simulink model "mud"  (Simulink 6.0)
settings: Solver=ode45  StartTime=0.0  StopTime=5000.0  RelTol=1e-3
undefined symbols (not defined in the file or in its folder): cputime
libraries: commsink2 x3
settings Model: LastModifiedBy=god

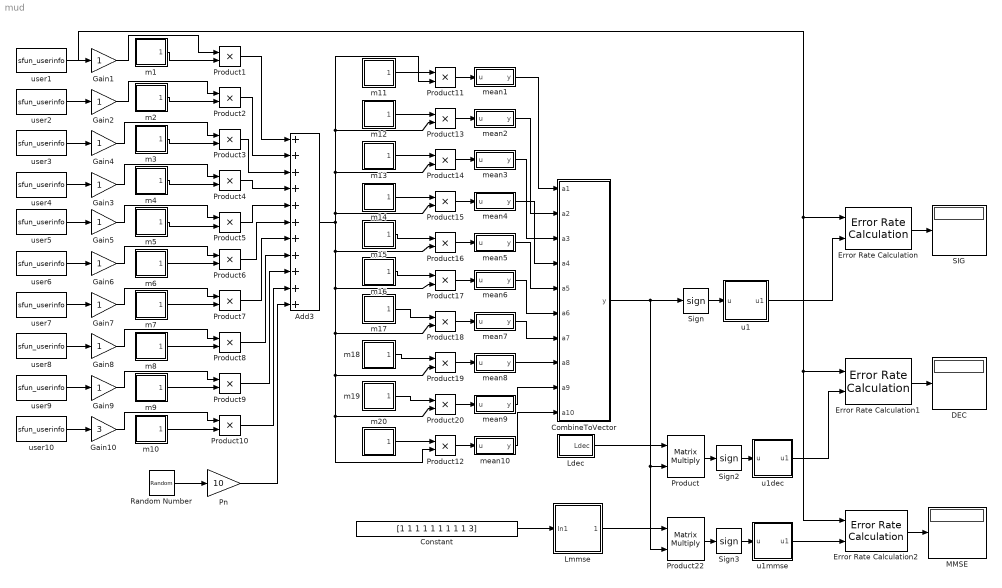
== system mud ==
  Add3 : Sum  Inputs=+++++++++++  OutScaling=2^-10  SampleTime=1
  CombineToVector : Stateflow chart
  Constant : Constant  Value=[1 1 1 1 1 1 1 1 1 3]
  DEC : Display
  Error Rate Calculation : commsink2/Error Rate Calculation  N=0  st_delay=0  cp_mode=Entire frame  subframe=[]  PMode=Port  WsName=ErrorVec  RsMode2=off  stop=off  numErr=100  maxBits=1e6
  Error Rate Calculation1 : commsink2/Error Rate Calculation  N=0  st_delay=0  cp_mode=Entire frame  subframe=[]  PMode=Port  WsName=ErrorVec  RsMode2=off  stop=off  numErr=100  maxBits=1e6
  Error Rate Calculation2 : commsink2/Error Rate Calculation  N=0  st_delay=0  cp_mode=Entire frame  subframe=[]  PMode=Port  WsName=ErrorVec  RsMode2=off  stop=off  numErr=100  maxBits=1e6
  Gain{1..9} (9 alike) : Gain  SampleTime=1
  Gain10 : Gain  Gain=3  SampleTime=1
  Ldec : Subsystem
  Lmmse : Subsystem
  MMSE : Display
  Pn : Gain  Gain=10  SampleTime=1
  Product : Product  Multiplication=Matrix(*)  RndMeth=Zero
  Product{1..20} (20 alike) : Product  SampleTime=1  RndMeth=Zero
  Product22 : Product  Multiplication=Matrix(*)  RndMeth=Zero
  Random Number : RandomNumber  Seed=cputime  SampleTime=1
  SIG : Display
  Sign : Signum
  Sign2 : Signum
  Sign3 : Signum
  m1 : Subsystem
  m10 : Subsystem
  m11 : Subsystem
  m12 : Subsystem
  m13 : Subsystem
  m14 : Subsystem
  m15 : Subsystem
  m16 : Subsystem
  m17 : Subsystem
  m18 : Subsystem
  m19 : Subsystem
  m2 : Subsystem
  m20 : Subsystem
  m3 : Subsystem
  m4 : Subsystem
  m5 : Subsystem
  m6 : Subsystem
  m7 : Subsystem
  m8 : Subsystem
  m9 : Subsystem
  mean1 : Stateflow chart
  mean10 : Stateflow chart
  mean2 : Stateflow chart
  mean3 : Stateflow chart
  mean4 : Stateflow chart
  mean5 : Stateflow chart
  mean6 : Stateflow chart
  mean7 : Stateflow chart
  mean8 : Stateflow chart
  mean9 : Stateflow chart
  u1 : Stateflow chart
  u1dec : Stateflow chart
  u1mmse : Stateflow chart
  user{1..10} (10 alike) : S-Function  FunctionName=sfun_userinfo
  wires:
  Gain1/1 -> Product1/1
  m1/1(Out1) -> Product1/2
  Gain2/1 -> Product2/1
  m2/1(Out1) -> Product2/2
  Gain4/1 -> Product3/1
  m3/1(Out1) -> Product3/2
  Gain3/1 -> Product4/1
  m4/1(Out1) -> Product4/2
  Gain5/1 -> Product5/1
  m5/1(Out1) -> Product5/2
  Gain6/1 -> Product6/1
  m6/1(Out1) -> Product6/2
  Gain7/1 -> Product7/1
  m7/1(Out1) -> Product7/2
  Gain8/1 -> Product8/1
  m8/1(Out1) -> Product8/2
  Gain9/1 -> Product9/1
  m9/1(Out1) -> Product9/2
  Gain10/1 -> Product10/1
  m10/1(Out1) -> Product10/2
  Random Number/1 -> Pn/1
  m11/1(Out1) -> Product11/1
  m12/1(Out1) -> Product13/1
  m13/1(Out1) -> Product14/1
  m14/1(Out1) -> Product15/1
  m15/1(Out1) -> Product16/1
  m16/1(Out1) -> Product17/1
  m17/1(Out1) -> Product18/1
  m18/1(Out1) -> Product19/1
  m20/1(Out1) -> Product12/1
  Add3/1 -> Product11/2, Product13/2, Product14/2, Product15/2, Product16/2, Product17/2, Product18/2, Product19/2, Product12/2, Product20/2
  Product13/1 -> mean2/1(u)
  Product14/1 -> mean3/1(u)
  Product15/1 -> mean4/1(u)
  Product16/1 -> mean5/1(u)
  Product17/1 -> mean6/1(u)
  Product18/1 -> mean7/1(u)
  Product19/1 -> mean8/1(u)
  Product20/1 -> mean9/1(u)
  Product12/1 -> mean10/1(u)
  Product11/1 -> mean1/1(u)
  mean1/1(y) -> CombineToVector/1(a1)
  mean2/1(y) -> CombineToVector/2(a2)
  mean3/1(y) -> CombineToVector/3(a3)
  mean4/1(y) -> CombineToVector/4(a4)
  mean5/1(y) -> CombineToVector/5(a5)
  mean6/1(y) -> CombineToVector/6(a6)
  mean7/1(y) -> CombineToVector/7(a7)
  mean9/1(y) -> CombineToVector/9(a9)
  mean10/1(y) -> CombineToVector/10(a10)
  CombineToVector/1(y) -> Product/2, Product22/2, Sign/1
  mean8/1(y) -> CombineToVector/8(a8)
  Product/1 -> Sign2/1
  user1/1 -> Gain1/1, Error Rate Calculation/1, Error Rate Calculation1/1, Error Rate Calculation2/1
  user2/1 -> Gain2/1
  user3/1 -> Gain4/1
  user4/1 -> Gain3/1
  user5/1 -> Gain5/1
  user6/1 -> Gain6/1
  user7/1 -> Gain7/1
  user8/1 -> Gain8/1
  user10/1 -> Gain10/1
  user9/1 -> Gain9/1
  Error Rate Calculation1/1 -> DEC/1
  Sign/1 -> u1/1(u)
  Sign2/1 -> u1dec/1(u)
  Sign3/1 -> u1mmse/1(u)
  u1/1(u1) -> Error Rate Calculation/2
  Product1/1 -> Add3/1
  Product2/1 -> Add3/2
  Product3/1 -> Add3/3
  Product4/1 -> Add3/4
  Product5/1 -> Add3/5
  Product6/1 -> Add3/6
  Product9/1 -> Add3/9
  Product10/1 -> Add3/10
  Product7/1 -> Add3/7
  Product8/1 -> Add3/8
  m19/1(Out1) -> Product20/1
  Product22/1 -> Sign3/1
  u1mmse/1(u1) -> Error Rate Calculation2/2
  u1dec/1(u1) -> Error Rate Calculation1/2
  Error Rate Calculation2/1 -> MMSE/1
  Error Rate Calculation/1 -> SIG/1
  Constant/1 -> Lmmse/1(In1)
  Lmmse/1(Lmmse) -> Product22/1
  Ldec/1(Ldec) -> Product/1
  Pn/1 -> Add3/11

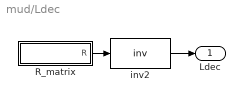
== system mud/Ldec ==
  R_matrix : Stateflow chart
  inv2 : MATLABFcn  MATLABFcn=inv  Output1D=off
  Ldec : Outport
  wires:
  R_matrix/1(R) -> inv2/1
  inv2/1 -> Ldec/1

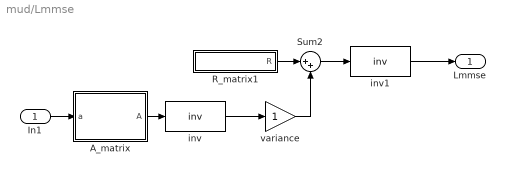
== system mud/Lmmse ==
  In1 : Inport  Port=1  LatchInput=off
  A_matrix : Stateflow chart
  R_matrix1 : Stateflow chart
  Sum2 : Sum  Inputs=|++
  inv : MATLABFcn  MATLABFcn=inv  Output1D=off
  inv1 : MATLABFcn  MATLABFcn=inv  Output1D=off
  variance : Gain
  Lmmse : Outport
  wires:
  A_matrix/1(A) -> inv/1
  inv/1 -> variance/1
  R_matrix1/1(R) -> Sum2/1
  variance/1 -> Sum2/2
  Sum2/1 -> inv1/1
  inv1/1 -> Lmmse/1
  In1/1 -> A_matrix/1(a)

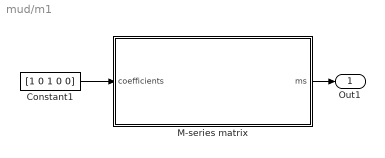
== system mud/m1 ==
  Constant1 : Constant  Value=[1 0 1 0 0]
  M-series matrix : Stateflow chart
  Out1 : Outport
  wires:
  Constant1/1 -> M-series matrix/1(coefficients)
  M-series matrix/1(ms) -> Out1/1

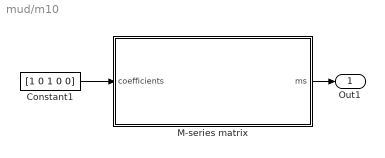
== system mud/m10 ==
  Constant1 : Constant  Value=[1 0 1 0 0]
  M-series matrix : Stateflow chart
  Out1 : Outport
  wires:
  Constant1/1 -> M-series matrix/1(coefficients)
  M-series matrix/1(ms) -> Out1/1

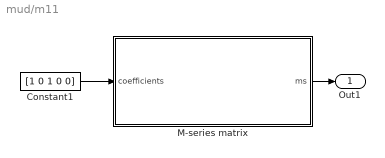
== system mud/m11 ==
  Constant1 : Constant  Value=[1 0 1 0 0]
  M-series matrix : Stateflow chart
  Out1 : Outport
  wires:
  M-series matrix/1(ms) -> Out1/1
  Constant1/1 -> M-series matrix/1(coefficients)

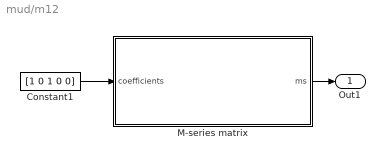
== system mud/m12 ==
  Constant1 : Constant  Value=[1 0 1 0 0]
  M-series matrix : Stateflow chart
  Out1 : Outport
  wires:
  M-series matrix/1(ms) -> Out1/1
  Constant1/1 -> M-series matrix/1(coefficients)

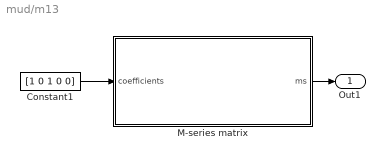
== system mud/m13 ==
  Constant1 : Constant  Value=[1 0 1 0 0]
  M-series matrix : Stateflow chart
  Out1 : Outport
  wires:
  M-series matrix/1(ms) -> Out1/1
  Constant1/1 -> M-series matrix/1(coefficients)

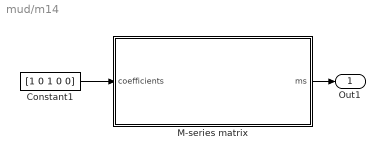
== system mud/m14 ==
  Constant1 : Constant  Value=[1 0 1 0 0]
  M-series matrix : Stateflow chart
  Out1 : Outport
  wires:
  M-series matrix/1(ms) -> Out1/1
  Constant1/1 -> M-series matrix/1(coefficients)

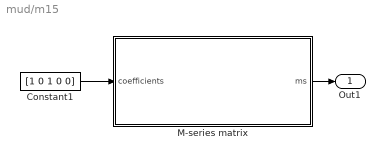
== system mud/m15 ==
  Constant1 : Constant  Value=[1 0 1 0 0]
  M-series matrix : Stateflow chart
  Out1 : Outport
  wires:
  M-series matrix/1(ms) -> Out1/1
  Constant1/1 -> M-series matrix/1(coefficients)

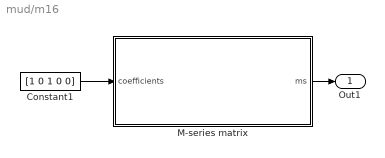
== system mud/m16 ==
  Constant1 : Constant  Value=[1 0 1 0 0]
  M-series matrix : Stateflow chart
  Out1 : Outport
  wires:
  M-series matrix/1(ms) -> Out1/1
  Constant1/1 -> M-series matrix/1(coefficients)

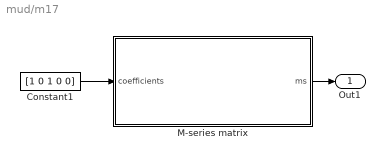
== system mud/m17 ==
  Constant1 : Constant  Value=[1 0 1 0 0]
  M-series matrix : Stateflow chart
  Out1 : Outport
  wires:
  M-series matrix/1(ms) -> Out1/1
  Constant1/1 -> M-series matrix/1(coefficients)

== system mud/m18 ==
  Constant1 : Constant  Value=[1 0 1 0 0]
  M-series matrix : Stateflow chart
  Out1 : Outport
  wires:
  M-series matrix/1(ms) -> Out1/1
  Constant1/1 -> M-series matrix/1(coefficients)

== system mud/m19 ==
  Constant1 : Constant  Value=[1 0 1 0 0]
  M-series matrix : Stateflow chart
  Out1 : Outport
  wires:
  M-series matrix/1(ms) -> Out1/1
  Constant1/1 -> M-series matrix/1(coefficients)

== system mud/m2 ==
  Constant1 : Constant  Value=[1 0 1 0 0]
  M-series matrix : Stateflow chart
  Out1 : Outport
  wires:
  Constant1/1 -> M-series matrix/1(coefficients)
  M-series matrix/1(ms) -> Out1/1

== system mud/m20 ==
  Constant1 : Constant  Value=[1 0 1 0 0]
  M-series matrix : Stateflow chart
  Out1 : Outport
  wires:
  M-series matrix/1(ms) -> Out1/1
  Constant1/1 -> M-series matrix/1(coefficients)

== system mud/m3 ==
  Constant1 : Constant  Value=[1 0 1 0 0]
  M-series matrix : Stateflow chart
  Out1 : Outport
  wires:
  Constant1/1 -> M-series matrix/1(coefficients)
  M-series matrix/1(ms) -> Out1/1

== system mud/m4 ==
  Constant1 : Constant  Value=[1 0 1 0 0]
  M-series matrix : Stateflow chart
  Out1 : Outport
  wires:
  Constant1/1 -> M-series matrix/1(coefficients)
  M-series matrix/1(ms) -> Out1/1

== system mud/m5 ==
  Constant1 : Constant  Value=[1 0 1 0 0]
  M-series matrix : Stateflow chart
  Out1 : Outport
  wires:
  Constant1/1 -> M-series matrix/1(coefficients)
  M-series matrix/1(ms) -> Out1/1

== system mud/m6 ==
  Constant1 : Constant  Value=[1 0 1 0 0]
  M-series matrix : Stateflow chart
  Out1 : Outport
  wires:
  Constant1/1 -> M-series matrix/1(coefficients)
  M-series matrix/1(ms) -> Out1/1

== system mud/m7 ==
  Constant1 : Constant  Value=[1 0 1 0 0]
  M-series matrix : Stateflow chart
  Out1 : Outport
  wires:
  Constant1/1 -> M-series matrix/1(coefficients)
  M-series matrix/1(ms) -> Out1/1

== system mud/m8 ==
  Constant1 : Constant  Value=[1 0 1 0 0]
  M-series matrix : Stateflow chart
  Out1 : Outport
  wires:
  Constant1/1 -> M-series matrix/1(coefficients)
  M-series matrix/1(ms) -> Out1/1

== system mud/m9 ==
  Constant1 : Constant  Value=[1 0 1 0 0]
  M-series matrix : Stateflow chart
  Out1 : Outport
  wires:
  Constant1/1 -> M-series matrix/1(coefficients)
  M-series matrix/1(ms) -> Out1/1

== matlab function m2/M-series matrix ==
  data: coefficients input inherited; ms output inherited
function ms = mseries(coefficients)
len=length(coefficients);
L=2^len-1;
registers=[zeros(1,len-1),1];
newregisters=zeros(1,len);
a=[0 0 0 0 0 0 0 0 0 0 0 0 0 0 0 0 0 0 0 0 0 0 0 0 0 0 0 0 0 0 0];
a(1)=registers(1);
for i= 2:L
    newregisters(1:len-1) = registers(2:len);
    newregisters(len) = mod(sum(coefficients.*registers'),2);
    registers=newregisters;
    a(i)=registers(1);
end
for j=1:L
    if a(j)==0
        a(j)=1;
    else
        a(j)=-1;
    end
end

atemp=zeros(31);
for p=1:L
  atemp(p,:)=a;
  temp=a(1);
  for q=1:L-1
  a(q)=a(q+1);
  end
  a(L)=temp;
end
ms=atemp(2,:);

== matlab function m3/M-series matrix ==
  data: coefficients input inherited; ms output inherited
function ms = mseries(coefficients)
len=length(coefficients);
L=2^len-1;
registers=[zeros(1,len-1),1];
newregisters=zeros(1,len);
a=[0 0 0 0 0 0 0 0 0 0 0 0 0 0 0 0 0 0 0 0 0 0 0 0 0 0 0 0 0 0 0];
a(1)=registers(1);
for i= 2:L
    newregisters(1:len-1) = registers(2:len);
    newregisters(len) = mod(sum(coefficients.*registers'),2);
    registers=newregisters;
    a(i)=registers(1);
end
for j=1:L
    if a(j)==0
        a(j)=1;
    else
        a(j)=-1;
    end
end

atemp=zeros(31);
for p=1:L
  atemp(p,:)=a;
  temp=a(1);
  for q=1:L-1
  a(q)=a(q+1);
  end
  a(L)=temp;
end
ms=atemp(3,:);

== matlab function m4/M-series matrix ==
  data: coefficients input inherited; ms output inherited
function ms = mseries(coefficients)
len=length(coefficients);
L=2^len-1;
registers=[zeros(1,len-1),1];
newregisters=zeros(1,len);
a=[0 0 0 0 0 0 0 0 0 0 0 0 0 0 0 0 0 0 0 0 0 0 0 0 0 0 0 0 0 0 0];
a(1)=registers(1);
for i= 2:L
    newregisters(1:len-1) = registers(2:len);
    newregisters(len) = mod(sum(coefficients.*registers'),2);
    registers=newregisters;
    a(i)=registers(1);
end
for j=1:L
    if a(j)==0
        a(j)=1;
    else
        a(j)=-1;
    end
end

atemp=zeros(31);
for p=1:L
  atemp(p,:)=a;
  temp=a(1);
  for q=1:L-1
  a(q)=a(q+1);
  end
  a(L)=temp;
end
ms=atemp(4,:);

== matlab function m5/M-series matrix ==
  data: coefficients input inherited; ms output inherited
function ms = mseries(coefficients)
len=length(coefficients);
L=2^len-1;
registers=[zeros(1,len-1),1];
newregisters=zeros(1,len);
a=[0 0 0 0 0 0 0 0 0 0 0 0 0 0 0 0 0 0 0 0 0 0 0 0 0 0 0 0 0 0 0];
a(1)=registers(1);
for i= 2:L
    newregisters(1:len-1) = registers(2:len);
    newregisters(len) = mod(sum(coefficients.*registers'),2);
    registers=newregisters;
    a(i)=registers(1);
end
for j=1:L
    if a(j)==0
        a(j)=1;
    else
        a(j)=-1;
    end
end

atemp=zeros(31);
for p=1:L
  atemp(p,:)=a;
  temp=a(1);
  for q=1:L-1
  a(q)=a(q+1);
  end
  a(L)=temp;
end
ms=atemp(5,:);

== matlab function m6/M-series matrix ==
  data: coefficients input inherited; ms output inherited
function ms = mseries(coefficients)
len=length(coefficients);
L=2^len-1;
registers=[zeros(1,len-1),1];
newregisters=zeros(1,len);
a=[0 0 0 0 0 0 0 0 0 0 0 0 0 0 0 0 0 0 0 0 0 0 0 0 0 0 0 0 0 0 0];
a(1)=registers(1);
for i= 2:L
    newregisters(1:len-1) = registers(2:len);
    newregisters(len) = mod(sum(coefficients.*registers'),2);
    registers=newregisters;
    a(i)=registers(1);
end
for j=1:L
    if a(j)==0
        a(j)=1;
    else
        a(j)=-1;
    end
end

atemp=zeros(31);
for p=1:L
  atemp(p,:)=a;
  temp=a(1);
  for q=1:L-1
  a(q)=a(q+1);
  end
  a(L)=temp;
end
ms=atemp(6,:);

== matlab function m7/M-series matrix ==
  data: coefficients input inherited; ms output inherited
function ms = mseries(coefficients)
len=length(coefficients);
L=2^len-1;
registers=[zeros(1,len-1),1];
newregisters=zeros(1,len);
a=[0 0 0 0 0 0 0 0 0 0 0 0 0 0 0 0 0 0 0 0 0 0 0 0 0 0 0 0 0 0 0];
a(1)=registers(1);
for i= 2:L
    newregisters(1:len-1) = registers(2:len);
    newregisters(len) = mod(sum(coefficients.*registers'),2);
    registers=newregisters;
    a(i)=registers(1);
end
for j=1:L
    if a(j)==0
        a(j)=1;
    else
        a(j)=-1;
    end
end

atemp=zeros(31);
for p=1:L
  atemp(p,:)=a;
  temp=a(1);
  for q=1:L-1
  a(q)=a(q+1);
  end
  a(L)=temp;
end
ms=atemp(7,:);

== matlab function m8/M-series matrix ==
  data: coefficients input inherited; ms output inherited
function ms = mseries(coefficients)
len=length(coefficients);
L=2^len-1;
registers=[zeros(1,len-1),1];
newregisters=zeros(1,len);
a=[0 0 0 0 0 0 0 0 0 0 0 0 0 0 0 0 0 0 0 0 0 0 0 0 0 0 0 0 0 0 0];
a(1)=registers(1);
for i= 2:L
    newregisters(1:len-1) = registers(2:len);
    newregisters(len) = mod(sum(coefficients.*registers'),2);
    registers=newregisters;
    a(i)=registers(1);
end
for j=1:L
    if a(j)==0
        a(j)=1;
    else
        a(j)=-1;
    end
end

atemp=zeros(31);
for p=1:L
  atemp(p,:)=a;
  temp=a(1);
  for q=1:L-1
  a(q)=a(q+1);
  end
  a(L)=temp;
end
ms=atemp(8,:);

== matlab function m9/M-series matrix ==
  data: coefficients input inherited; ms output inherited
function ms = mseries(coefficients)
len=length(coefficients);
L=2^len-1;
registers=[zeros(1,len-1),1];
newregisters=zeros(1,len);
a=[0 0 0 0 0 0 0 0 0 0 0 0 0 0 0 0 0 0 0 0 0 0 0 0 0 0 0 0 0 0 0];
a(1)=registers(1);
for i= 2:L
    newregisters(1:len-1) = registers(2:len);
    newregisters(len) = mod(sum(coefficients.*registers'),2);
    registers=newregisters;
    a(i)=registers(1);
end
for j=1:L
    if a(j)==0
        a(j)=1;
    else
        a(j)=-1;
    end
end

atemp=zeros(31);
for p=1:L
  atemp(p,:)=a;
  temp=a(1);
  for q=1:L-1
  a(q)=a(q+1);
  end
  a(L)=temp;
end
ms=atemp(9,:);

== matlab function m10/M-series matrix ==
  data: coefficients input inherited; ms output inherited
function ms = mseries(coefficients)
len=length(coefficients);
L=2^len-1;
registers=[zeros(1,len-1),1];
newregisters=zeros(1,len);
a=[0 0 0 0 0 0 0 0 0 0 0 0 0 0 0 0 0 0 0 0 0 0 0 0 0 0 0 0 0 0 0];
a(1)=registers(1);
for i= 2:L
    newregisters(1:len-1) = registers(2:len);
    newregisters(len) = mod(sum(coefficients.*registers'),2);
    registers=newregisters;
    a(i)=registers(1);
end
for j=1:L
    if a(j)==0
        a(j)=1;
    else
        a(j)=-1;
    end
end

atemp=zeros(31);
for p=1:L
  atemp(p,:)=a;
  temp=a(1);
  for q=1:L-1
  a(q)=a(q+1);
  end
  a(L)=temp;
end
ms=atemp(10,:);

== matlab function m11/M-series matrix ==
  data: coefficients input inherited; ms output inherited
function ms = mseries(coefficients)
len=length(coefficients);
L=2^len-1;
registers=[zeros(1,len-1),1];
newregisters=zeros(1,len);
a=[0 0 0 0 0 0 0 0 0 0 0 0 0 0 0 0 0 0 0 0 0 0 0 0 0 0 0 0 0 0 0];
a(1)=registers(1);
for i= 2:L
    newregisters(1:len-1) = registers(2:len);
    newregisters(len) = mod(sum(coefficients.*registers'),2);
    registers=newregisters;
    a(i)=registers(1);
end
for j=1:L
    if a(j)==0
        a(j)=1;
    else
        a(j)=-1;
    end
end

atemp=zeros(31);
for p=1:L
  atemp(p,:)=a;
  temp=a(1);
  for q=1:L-1
  a(q)=a(q+1);
  end
  a(L)=temp;
end
ms=atemp(1,:);

== matlab function m12/M-series matrix ==
  data: coefficients input inherited; ms output inherited
function ms = mseries(coefficients)
len=length(coefficients);
L=2^len-1;
registers=[zeros(1,len-1),1];
newregisters=zeros(1,len);
a=[0 0 0 0 0 0 0 0 0 0 0 0 0 0 0 0 0 0 0 0 0 0 0 0 0 0 0 0 0 0 0];
a(1)=registers(1);
for i= 2:L
    newregisters(1:len-1) = registers(2:len);
    newregisters(len) = mod(sum(coefficients.*registers'),2);
    registers=newregisters;
    a(i)=registers(1);
end
for j=1:L
    if a(j)==0
        a(j)=1;
    else
        a(j)=-1;
    end
end

atemp=zeros(31);
for p=1:L
  atemp(p,:)=a;
  temp=a(1);
  for q=1:L-1
  a(q)=a(q+1);
  end
  a(L)=temp;
end
ms=atemp(2,:);

== matlab function m13/M-series matrix ==
  data: coefficients input inherited; ms output inherited
function ms = mseries(coefficients)
len=length(coefficients);
L=2^len-1;
registers=[zeros(1,len-1),1];
newregisters=zeros(1,len);
a=[0 0 0 0 0 0 0 0 0 0 0 0 0 0 0 0 0 0 0 0 0 0 0 0 0 0 0 0 0 0 0];
a(1)=registers(1);
for i= 2:L
    newregisters(1:len-1) = registers(2:len);
    newregisters(len) = mod(sum(coefficients.*registers'),2);
    registers=newregisters;
    a(i)=registers(1);
end
for j=1:L
    if a(j)==0
        a(j)=1;
    else
        a(j)=-1;
    end
end

atemp=zeros(31);
for p=1:L
  atemp(p,:)=a;
  temp=a(1);
  for q=1:L-1
  a(q)=a(q+1);
  end
  a(L)=temp;
end
ms=atemp(3,:);

== matlab function m14/M-series matrix ==
  data: coefficients input inherited; ms output inherited
function ms = mseries(coefficients)
len=length(coefficients);
L=2^len-1;
registers=[zeros(1,len-1),1];
newregisters=zeros(1,len);
a=[0 0 0 0 0 0 0 0 0 0 0 0 0 0 0 0 0 0 0 0 0 0 0 0 0 0 0 0 0 0 0];
a(1)=registers(1);
for i= 2:L
    newregisters(1:len-1) = registers(2:len);
    newregisters(len) = mod(sum(coefficients.*registers'),2);
    registers=newregisters;
    a(i)=registers(1);
end
for j=1:L
    if a(j)==0
        a(j)=1;
    else
        a(j)=-1;
    end
end

atemp=zeros(31);
for p=1:L
  atemp(p,:)=a;
  temp=a(1);
  for q=1:L-1
  a(q)=a(q+1);
  end
  a(L)=temp;
end
ms=atemp(4,:);

== matlab function m15/M-series matrix ==
  data: coefficients input inherited; ms output inherited
function ms = mseries(coefficients)
len=length(coefficients);
L=2^len-1;
registers=[zeros(1,len-1),1];
newregisters=zeros(1,len);
a=[0 0 0 0 0 0 0 0 0 0 0 0 0 0 0 0 0 0 0 0 0 0 0 0 0 0 0 0 0 0 0];
a(1)=registers(1);
for i= 2:L
    newregisters(1:len-1) = registers(2:len);
    newregisters(len) = mod(sum(coefficients.*registers'),2);
    registers=newregisters;
    a(i)=registers(1);
end
for j=1:L
    if a(j)==0
        a(j)=1;
    else
        a(j)=-1;
    end
end

atemp=zeros(31);
for p=1:L
  atemp(p,:)=a;
  temp=a(1);
  for q=1:L-1
  a(q)=a(q+1);
  end
  a(L)=temp;
end
ms=atemp(5,:);

== matlab function m16/M-series matrix ==
  data: coefficients input inherited; ms output inherited
function ms = mseries(coefficients)
len=length(coefficients);
L=2^len-1;
registers=[zeros(1,len-1),1];
newregisters=zeros(1,len);
a=[0 0 0 0 0 0 0 0 0 0 0 0 0 0 0 0 0 0 0 0 0 0 0 0 0 0 0 0 0 0 0];
a(1)=registers(1);
for i= 2:L
    newregisters(1:len-1) = registers(2:len);
    newregisters(len) = mod(sum(coefficients.*registers'),2);
    registers=newregisters;
    a(i)=registers(1);
end
for j=1:L
    if a(j)==0
        a(j)=1;
    else
        a(j)=-1;
    end
end

atemp=zeros(31);
for p=1:L
  atemp(p,:)=a;
  temp=a(1);
  for q=1:L-1
  a(q)=a(q+1);
  end
  a(L)=temp;
end
ms=atemp(6,:);

== matlab function m17/M-series matrix ==
  data: coefficients input inherited; ms output inherited
function ms = mseries(coefficients)
len=length(coefficients);
L=2^len-1;
registers=[zeros(1,len-1),1];
newregisters=zeros(1,len);
a=[0 0 0 0 0 0 0 0 0 0 0 0 0 0 0 0 0 0 0 0 0 0 0 0 0 0 0 0 0 0 0];
a(1)=registers(1);
for i= 2:L
    newregisters(1:len-1) = registers(2:len);
    newregisters(len) = mod(sum(coefficients.*registers'),2);
    registers=newregisters;
    a(i)=registers(1);
end
for j=1:L
    if a(j)==0
        a(j)=1;
    else
        a(j)=-1;
    end
end

atemp=zeros(31);
for p=1:L
  atemp(p,:)=a;
  temp=a(1);
  for q=1:L-1
  a(q)=a(q+1);
  end
  a(L)=temp;
end
ms=atemp(7,:);

== matlab function m18/M-series matrix ==
  data: coefficients input inherited; ms output inherited
function ms = mseries(coefficients)
len=length(coefficients);
L=2^len-1;
registers=[zeros(1,len-1),1];
newregisters=zeros(1,len);
a=[0 0 0 0 0 0 0 0 0 0 0 0 0 0 0 0 0 0 0 0 0 0 0 0 0 0 0 0 0 0 0];
a(1)=registers(1);
for i= 2:L
    newregisters(1:len-1) = registers(2:len);
    newregisters(len) = mod(sum(coefficients.*registers'),2);
    registers=newregisters;
    a(i)=registers(1);
end
for j=1:L
    if a(j)==0
        a(j)=1;
    else
        a(j)=-1;
    end
end

atemp=zeros(31);
for p=1:L
  atemp(p,:)=a;
  temp=a(1);
  for q=1:L-1
  a(q)=a(q+1);
  end
  a(L)=temp;
end
ms=atemp(8,:);

== matlab function m19/M-series matrix ==
  data: coefficients input inherited; ms output inherited
function ms = mseries(coefficients)
len=length(coefficients);
L=2^len-1;
registers=[zeros(1,len-1),1];
newregisters=zeros(1,len);
a=[0 0 0 0 0 0 0 0 0 0 0 0 0 0 0 0 0 0 0 0 0 0 0 0 0 0 0 0 0 0 0];
a(1)=registers(1);
for i= 2:L
    newregisters(1:len-1) = registers(2:len);
    newregisters(len) = mod(sum(coefficients.*registers'),2);
    registers=newregisters;
    a(i)=registers(1);
end
for j=1:L
    if a(j)==0
        a(j)=1;
    else
        a(j)=-1;
    end
end

atemp=zeros(31);
for p=1:L
  atemp(p,:)=a;
  temp=a(1);
  for q=1:L-1
  a(q)=a(q+1);
  end
  a(L)=temp;
end
ms=atemp(9,:);

== matlab function m20/M-series matrix ==
  data: coefficients input inherited; ms output inherited
function ms = mseries(coefficients)
len=length(coefficients);
L=2^len-1;
registers=[zeros(1,len-1),1];
newregisters=zeros(1,len);
a=[0 0 0 0 0 0 0 0 0 0 0 0 0 0 0 0 0 0 0 0 0 0 0 0 0 0 0 0 0 0 0];
a(1)=registers(1);
for i= 2:L
    newregisters(1:len-1) = registers(2:len);
    newregisters(len) = mod(sum(coefficients.*registers'),2);
    registers=newregisters;
    a(i)=registers(1);
end
for j=1:L
    if a(j)==0
        a(j)=1;
    else
        a(j)=-1;
    end
end

atemp=zeros(31);
for p=1:L
  atemp(p,:)=a;
  temp=a(1);
  for q=1:L-1
  a(q)=a(q+1);
  end
  a(L)=temp;
end
ms=atemp(10,:);

== matlab function mean2 ==
  data: u input inherited; y output inherited
function y = mean(u)
y = mean(u);

== matlab function mean3 ==
  data: u input inherited; y output inherited
function y = mean(u)
y = mean(u);

== matlab function mean1 ==
  data: u input inherited; y output inherited
function y = mean(u)
y = mean(u);

== matlab function mean4 ==
  data: u input inherited; y output inherited
function y = mean(u)
y = mean(u);

== matlab function mean5 ==
  data: u input inherited; y output inherited
function y = mean(u)
y = mean(u);

== matlab function mean6 ==
  data: u input inherited; y output inherited
function y = mean(u)
y = mean(u);

== matlab function mean7 ==
  data: u input inherited; y output inherited
function y = mean(u)
y = mean(u);

== matlab function mean8 ==
  data: u input inherited; y output inherited
function y = mean(u)
y = mean(u);

== matlab function mean9 ==
  data: u input inherited; y output inherited
function y = mean(u)
y = mean(u);

== matlab function mean10 ==
  data: u input inherited; y output inherited
function y = mean(u)
y = mean(u);

== matlab function Ldec/R_matrix ==
  data: R output inherited
function R = R_matrix()
R=(ones(10)+(31-1)*eye(10))/31;

== matlab function Lmmse/R_matrix1 ==
  data: R output inherited
function R = R_matrix()
R=(ones(10)+(31-1)*eye(10))/31;

== matlab function Lmmse/A_matrix ==
  data: a input inherited; A output inherited
function A = A(a)
A=diag(a);

== matlab function u1 ==
  data: u1 output inherited; u input inherited
function u1=fcn(u)
u1=u(1);

== matlab function u1dec ==
  data: u1 output inherited; u input inherited
function u1=fcn(u)
u1=u(1);

== matlab function m1/M-series matrix ==
  data: coefficients input inherited; ms output inherited
function ms = mseries(coefficients)
len=length(coefficients);
L=2^len-1;
registers=[zeros(1,len-1),1];
newregisters=zeros(1,len);
a=[0 0 0 0 0 0 0 0 0 0 0 0 0 0 0 0 0 0 0 0 0 0 0 0 0 0 0 0 0 0 0];
a(1)=registers(1);
for i= 2:L
    newregisters(1:len-1) = registers(2:len);
    newregisters(len) = mod(sum(coefficients.*registers'),2);
    registers=newregisters;
    a(i)=registers(1);
end
for j=1:L
    if a(j)==0
        a(j)=1;
    else
        a(j)=-1;
    end
end

atemp=zeros(31);
for p=1:L
  atemp(p,:)=a;
  temp=a(1);
  for q=1:L-1
  a(q)=a(q+1);
  end
  a(L)=temp;
end
ms=atemp(1,:);

== matlab function u1mmse ==
  data: u1 output inherited; u input inherited
function u1=fcn(u)
u1=u(1);

== matlab function CombineToVector ==
  data: a1 input inherited; y output inherited; a2 input inherited; a3 input inherited; a4 input inherited; a5 input inherited; a6 input inherited; a7 input inherited; a8 input inherited; a9 input inherited; a10 input inherited
function y =y1(a1,a2,a3,a4,a5,a6,a7,a8,a9,a10)

y = [a1,a2,a3,a4,a5,a6,a7,a8,a9,a10]';
